simulink model "cp_wideband_gammatone_filter"  (R2020b)
settings: Solver=FixedStepDiscrete  StartTime=0.0  StopTime=stopTime  FixedStep=2.0833333333333333e-05  RelTol=1e-3
values from neighbouring files (symbols this model uses):
  cf = 1000    [modelparameters.m]
  cordiciterationswb = 52    [modelparameters.m]
  delta_phase = -TWOPI*centerfreq*tdres    [modelparameters.m]
  TauWBMax = 0.000163019356301846    (= 0.000163019356302)    [modelparameters.m]
  tdres = 1/Fs    (= 2.08333333333e-05)    [modelparameters.m]
  wborder = 3    [modelparameters.m]
undefined symbols (not defined in the file or in its folder): jsin
settings Model: Creator=Ross  LastModifiedBy=tyler
settings DataIOCC: SaveOutput=off  SaveTime=off  ReturnWorkspaceOutputs=off
settings OptimizationCC: BlockReduction=off  ConditionallyExecuteInputs=off  DefaultParameterBehavior=Inlined
settings DebuggingCC: ReadBeforeWriteMsg=DisableAll  WriteAfterWriteMsg=DisableAll  WriteAfterReadMsg=DisableAll  AlgebraicLoopMsg=error  MultiTaskDSMMsg=none  SingleTaskRateTransMsg=error  PregeneratedLibrarySubsystemCodeDiagnostic=none  ArithmeticOperatorsInVariantConditions=warning
settings HardwareCC: ProdBitPerPointer=32  ProdBitPerSizeT=32  ProdBitPerPtrDiffT=32  ProdLargestAtomicFloat=None  ProdIntDivRoundTo=Undefined  ProdEndianess=Unspecified  ProdWordSize=32  ProdHWDeviceType=ASIC/FPGA->ASIC/FPGA  TargetBitPerPointer=64  TargetBitPerSizeT=64  TargetBitPerPtrDiffT=64  TargetLongLongMode=on  TargetIntDivRoundTo=Zero  TargetEndianess=LittleEndian  TargetWordSize=64  TargetHWDeviceType=Custom Processor->MATLAB Host Computer  ProdEqTarget=off
settings ModelReferenceCC: UpdateModelReferenceTargets=IfOutOfDate  ModelReferenceNumInstancesAllowed=Single
settings SFSimCC: SFSimEcho=off  SimUseLocalCustomCode=off  CustomCodeUndefinedFunction=UseInterfaceOnly
settings RTWCC: RTWUseLocalCustomCode=off

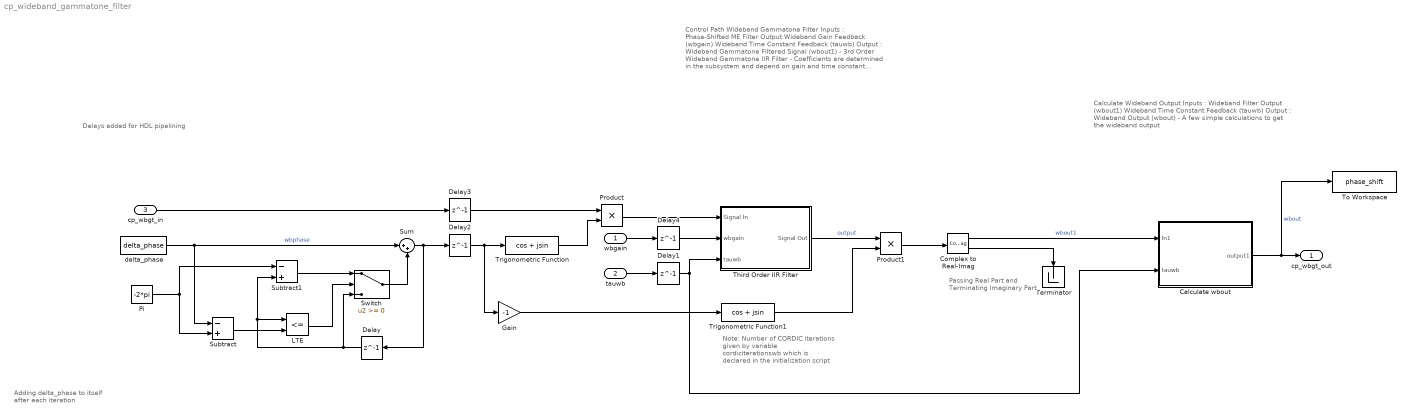
== system cp_wideband_gammatone_filter ==
  note: Calculate Wideband Output
      |
      | Inputs : Wideband Filter Output (wbout1)
      | Wideband Time Constant Feedback (tauwb)
      |
      | Output : Wideband Output (wbout)
      |
      | - A few simple calculations to get the wideband output
  note: Control Path Wideband Gammatone Filter
      |
      | Inputs : Phase-Shifted ME Filter Output
      | Wideband Gain Feedback (wbgain)
      | Wideband Time Constant Feedback (tauwb)
      |
      | Output : Wideband Gammatone Filtered Signal (wbout1)
      |
      | - 3rd Order Wideband Gammatone IIR Filter
      |
      | - Coefficients are determined in the subsystem and depend on gain and time constant feedback
      |
      | - Implemented w/ Direct Form I Block Structure
  note: Adding delta_phase to itself after each iteration
  note: Note: Number of CORDIC iterations given by variable cordiciterationswb which is declared in the initialization script
  note: Passing Real Part and Terminating Imaginary Part
  note: Delays added for HDL pipelining
  wbgain : Inport  OutDataTypeStr=single  PortDimensions=1  SampleTime=[2.0833333333333333e-05,0]
  tauwb : Inport  Port=2  OutDataTypeStr=single  PortDimensions=1  SampleTime=[2.0833333333333333e-05,0]
  cp_wbgt_in : Inport  Port=3  OutDataTypeStr=single  PortDimensions=1  SampleTime=[2.0833333333333333e-05,0]
  Calculate wbout : Subsystem
  Complex to Real-Imag : ComplexToRealImag
  Delay{,1..4} (5 alike) : Delay  DelayLength=1  InitialCondition=0  UseCircularBuffer=on
  Gain : Gain  Gain=-1  OutDataTypeStr=single
  LTE : RelationalOperator  Operator=<=  OutDataTypeStr=boolean  RndMeth=Simplest
  Pi : Constant  Value=-2*pi  OutDataTypeStr=Inherit: Inherit via back propagation  SampleTime=-1
  Product : Product  OutDataTypeStr=single
  Product1 : Product  OutDataTypeStr=single
  Subtract : Sum  Inputs=-+
  Subtract1 : Sum  Inputs=-+
  Sum : Sum  Inputs=|++
  Switch : Switch
  Terminator : Terminator
  Third Order IIR Filter : Subsystem
  To Workspace : ToWorkspace  VariableName=phase_shift  SaveFormat=Timeseries  SampleTime=-1
  Trigonometric Function : Trigonometry  Operator=cos + jsin  NumberOfIterations=cordiciterationswb
  Trigonometric Function1 : Trigonometry  Operator=cos + jsin  NumberOfIterations=cordiciterationswb
  delta_phase : Constant  Value=delta_phase  OutDataTypeStr=single  SampleTime=-1
  cp_wbgt_out : Outport  OutDataTypeStr=single  PortDimensions=1  SampleTime=[2.0833333333333333e-05,0]  VectorParamsAs1DForOutWhenUnconnected=off
  wires:
  Trigonometric Function1/1 -> Product1/2
  Gain/1 -> Trigonometric Function1/1
  Complex to Real-Imag/2 -> Terminator/1
  Product1/1 -> Complex to Real-Imag/1
  Product/1 -> Third Order IIR Filter/1(Signal In)
  Trigonometric Function/1 -> Product/2
  Third Order IIR Filter/1(Signal Out) -> Product1/1  "output"
  Complex to Real-Imag/1 -> Calculate wbout/1(In1)  "wbout1"
  Calculate wbout/1(output1) -> To Workspace/1, cp_wbgt_out/1  "wbout"
  delta_phase/1 -> Sum/1, Subtract/1  "wbphase"
  Subtract1/1 -> Switch/1
  Pi/1 -> Subtract/2, Subtract1/1
  LTE/1 -> Switch/2
  Delay/1 -> LTE/1, Subtract1/2, Switch/3
  Subtract/1 -> LTE/2
  Switch/1 -> Sum/2
  cp_wbgt_in/1 -> Delay3/1
  tauwb/1 -> Delay1/1
  wbgain/1 -> Delay4/1
  Sum/1 -> Delay2/1, Delay/1
  Delay2/1 -> Gain/1, Trigonometric Function/1
  Delay3/1 -> Product/1
  Delay1/1 -> Calculate wbout/2(tauwb), Third Order IIR Filter/3(tauwb)
  Delay4/1 -> Third Order IIR Filter/2(wbgain)

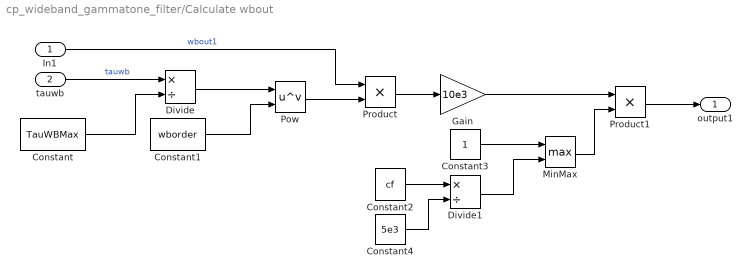
== system cp_wideband_gammatone_filter/Calculate wbout ==
  In1 : Inport
  tauwb : Inport  Port=2
  Constant : Constant  Value=TauWBMax  OutDataTypeStr=single  SampleTime=-1
  Constant1 : Constant  Value=wborder  OutDataTypeStr=single  SampleTime=-1
  Constant2 : Constant  Value=cf  OutDataTypeStr=single  SampleTime=-1
  Constant3 : Constant  OutDataTypeStr=single  SampleTime=-1
  Constant4 : Constant  Value=5e3  OutDataTypeStr=single  SampleTime=-1
  Divide : Product  Inputs=*/  RndMeth=Zero  SaturateOnIntegerOverflow=on
  Divide1 : Product  Inputs=*/  RndMeth=Zero  SaturateOnIntegerOverflow=on
  Gain : Gain  Gain=10e3
  MinMax : MinMax  Function=max  Inputs=2
  Pow : Math  Operator=pow  SignedPower=on  RndMeth=Zero  SaturateOnIntegerOverflow=on
  Product : Product
  Product1 : Product
  output1 : Outport  VectorParamsAs1DForOutWhenUnconnected=off
  wires:
  Constant4/1 -> Divide1/2
  Constant2/1 -> Divide1/1
  Product1/1 -> output1/1
  MinMax/1 -> Product1/2
  Constant3/1 -> MinMax/1
  Divide1/1 -> MinMax/2
  Gain/1 -> Product1/1
  Product/1 -> Gain/1
  Pow/1 -> Product/2
  Constant1/1 -> Pow/2
  Divide/1 -> Pow/1
  Constant/1 -> Divide/2
  In1/1 -> Product/1  "wbout1"
  tauwb/1 -> Divide/1  "tauwb"

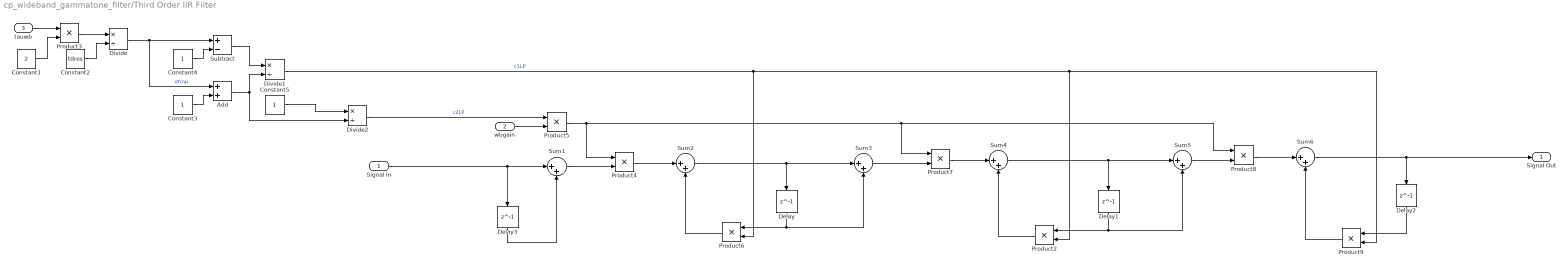
== system cp_wideband_gammatone_filter/Third Order IIR Filter ==
  Signal In : Inport
  wbgain : Inport  Port=2
  tauwb : Inport  Port=3
  Add : Sum
  Constant1 : Constant  Value=2  OutDataTypeStr=single  SampleTime=-1
  Constant2 : Constant  Value=tdres  OutDataTypeStr=single  SampleTime=-1
  Constant3 : Constant  OutDataTypeStr=single  SampleTime=-1
  Constant4 : Constant  OutDataTypeStr=single  SampleTime=-1
  Constant5 : Constant  OutDataTypeStr=single  SampleTime=-1
  Delay{,1..3} (4 alike) : Delay  DelayLength=1
  Divide : Product  Inputs=*/  RndMeth=Zero  SaturateOnIntegerOverflow=on
  Divide1 : Product  Inputs=*/  RndMeth=Zero  SaturateOnIntegerOverflow=on
  Divide2 : Product  Inputs=*/  RndMeth=Zero  SaturateOnIntegerOverflow=on
  Product{2..9} (8 alike) : Product
  Subtract : Sum  Inputs=+-
  Sum{1..6} (6 alike) : Sum  Inputs=|++
  Signal Out : Outport  VectorParamsAs1DForOutWhenUnconnected=off
  wires:
  Sum6/1 -> Delay2/1, Signal Out/1
  Product8/1 -> Sum6/1
  Subtract/1 -> Divide1/1
  Product2/1 -> Sum4/2
  Signal In/1 -> Delay3/1, Sum1/1
  Product5/1 -> Product4/1, Product7/1, Product8/1
  Constant1/1 -> Product3/2
  Divide2/1 -> Product5/1  "c2LP"
  Delay3/1 -> Sum1/2
  Divide/1 -> Add/1, Subtract/1  "dtmp"
  Sum3/1 -> Product7/2
  Add/1 -> Divide2/2, Divide1/2
  Sum5/1 -> Product8/2
  Delay/1 -> Sum3/2, Product6/1
  Constant5/1 -> Divide2/1
  Product7/1 -> Sum4/1
  Product9/1 -> Sum6/2
  Delay1/1 -> Sum5/2, Product2/1
  Sum2/1 -> Delay/1, Sum3/1
  Product6/1 -> Sum2/2
  Sum4/1 -> Delay1/1, Sum5/1
  tauwb/1 -> Product3/1
  Product3/1 -> Divide/1
  Constant4/1 -> Subtract/2
  wbgain/1 -> Product5/2
  Delay2/1 -> Product9/1
  Product4/1 -> Sum2/1
  Constant2/1 -> Divide/2
  Sum1/1 -> Product4/2
  Constant3/1 -> Add/2
  Divide1/1 -> Product6/2, Product9/2, Product2/2  "c1LP"
